simulink model "PID_controller"  (R2020b)
settings: Solver=ode45  StartTime=0.0  StopTime=10.0  RelTol=1e-3
settings Model: Creator=Lenovo  LastModifiedBy=Lenovo
settings DataIOCC: SaveOutput=off  SaveTime=off

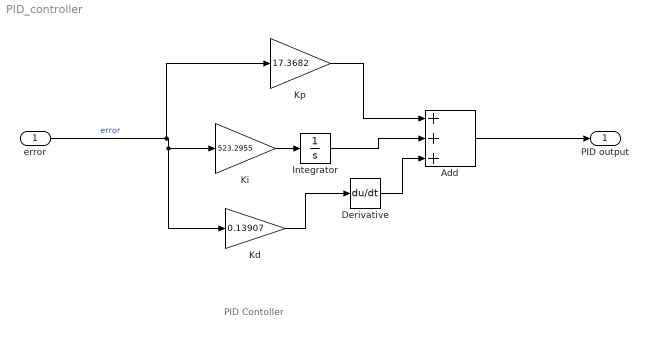
== system PID_controller ==
  note: PID Contoller
  error : Inport  OutDataTypeStr=double  PortDimensions=1  SampleTime=0
  Add : Sum  Inputs=+++
  Derivative : Derivative
  Integrator : Integrator
  Kd : Gain  Gain=0.13907
  Ki : Gain  Gain=523.2955
  Kp : Gain  Gain=17.3682
  PID output : Outport  OutDataTypeStr=double  PortDimensions=1  SampleTime=0
  wires:
  Integrator/1 -> Add/2
  error/1 -> Kd/1, Ki/1, Kp/1  "error"
  Kp/1 -> Add/1
  Ki/1 -> Integrator/1
  Add/1 -> PID output/1
  Kd/1 -> Derivative/1
  Derivative/1 -> Add/3
